simulink library "PropulsionModel"  (R2021b)
settings: Solver=VariableStepAuto  StartTime=0.0  StopTime=10.0  RelTol=1e-3
undefined symbols (not defined in the file or in its folder): eta_T_deg, n_rho, n_v, rho_ref_kgpm3, T_max_N, V_ref_mps
settings Model: Creator=setup  LastModifiedBy=dmgp1

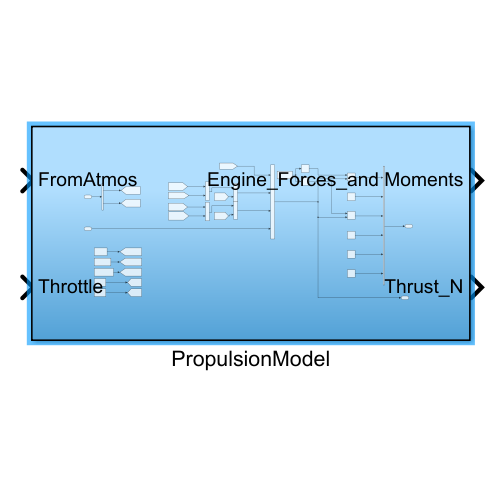
[thumbnail: Simulink's stored preview of the top-level diagram]
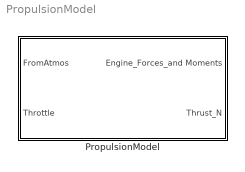
== system PropulsionModel ==
  PropulsionModel : Subsystem

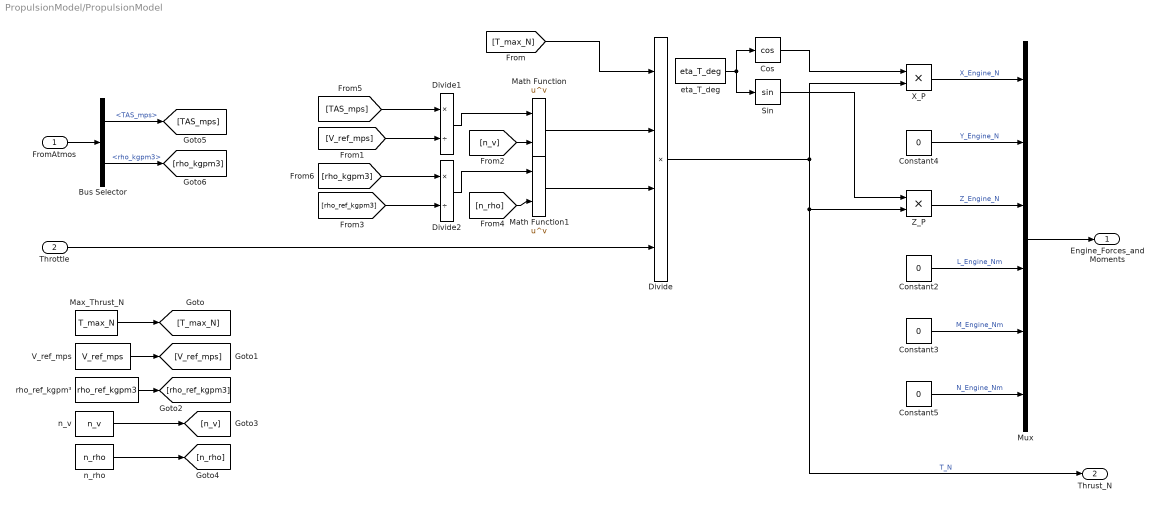
== system PropulsionModel/PropulsionModel ==
  FromAtmos : Inport
  Throttle : Inport  Port=2
  Bus Selector : BusSelector  OutputSignals=TAS_mps,rho_kgpm3
  Constant{2..5} (4 alike) : Constant  Value=0
  Cos : Trigonometry  Operator=cos
  Divide : Product  Inputs=****
  Divide1 : Product  Inputs=*/
  Divide2 : Product  Inputs=*/
  Math Function : Math  Operator=pow  OutMax=[1]  SaturateOnIntegerOverflow=on
  Math Function1 : Math  Operator=pow  OutMax=[1]  SaturateOnIntegerOverflow=on
  Max_Thrust_N : Constant  Value=T_max_N
  Mux : Mux  Inputs=6
  Sin : Trigonometry
  V_ref_mps : Constant  Value=V_ref_mps
  X_P : Product  Inputs=**
  Z_P : Product  Inputs=**
  eta_T_deg : Constant  Value=eta_T_deg
  n_rho : Constant  Value=n_rho
  n_v : Constant  Value=n_v
  rho_ref_kgpm³ : Constant  Value=rho_ref_kgpm3
  Engine_Forces_and Moments : Outport
  Thrust_N : Outport  Port=2
  wires:
  FromAtmos/1 -> Bus Selector/1
  Constant3/1 -> Mux/5  "M_Engine_Nm"
  Bus Selector/2 -> [rho_kgpm3]  "<rho_kgpm3>"
  Z_P/1 -> Mux/3  "Z_Engine_N"
  X_P/1 -> Mux/1  "X_Engine_N"
  Bus Selector/1 -> [TAS_mps]  "<TAS_mps>"
  Constant4/1 -> Mux/2  "Y_Engine_N"
  Mux/1 -> Engine_Forces_and Moments/1
  Constant2/1 -> Mux/4  "L_Engine_Nm"
  Constant5/1 -> Mux/6  "N_Engine_Nm"
  Divide/1 -> Thrust_N/1, Z_P/2, X_P/2  "T_N"
  Sin/1 -> Z_P/1
  Cos/1 -> X_P/1
  rho_ref_kgpm³/1 -> [rho_ref_kgpm3]
  Throttle/1 -> Divide/4
  Divide2/1 -> Math Function1/1
  [rho_ref_kgpm3] -> Divide2/2
  [T_max_N] -> Divide/1
  [TAS_mps] -> Divide1/1
  eta_T_deg/1 -> Cos/1, Sin/1
  n_rho/1 -> [n_rho]
  n_v/1 -> [n_v]
  Max_Thrust_N/1 -> [T_max_N]
  [n_v] -> Math Function/2
  [rho_kgpm3] -> Divide2/1
  [V_ref_mps] -> Divide1/2
  Math Function/1 -> Divide/2
  [n_rho] -> Math Function1/2
  V_ref_mps/1 -> [V_ref_mps]
  Divide1/1 -> Math Function/1
  Math Function1/1 -> Divide/3
